simulink model "autosar_bsw_simulation"  (R2022b)
settings: Solver=VariableStepAuto  StartTime=0.0  StopTime=10.0  RelTol=1e-3
libraries: autosarlibdem x1, autosarlibnvm x1, simulink x1
settings Model: Creator=The MathWorks, Inc.  LastModifiedBy=The MathWorks, Inc.
settings SolverCC: AlgebraicLoopSolver=TrustRegion
settings DataIOCC: ReturnWorkspaceOutputs=off
settings DebuggingCC: UnconnectedInputMsg=warning  UnconnectedOutputMsg=warning  UnconnectedLineMsg=warning  PregeneratedLibrarySubsystemCodeDiagnostic=none  SFMachineParentedDataDiag=warning  ArithmeticOperatorsInVariantConditions=warning
settings ModelReferenceCC: EnableRefExpFcnMdlSchedulingChecks=on
settings SFSimCC: SimUseLocalCustomCode=off  CustomCodeUndefinedFunction=UseInterfaceOnly
settings RTWCC: RTWUseLocalCustomCode=off

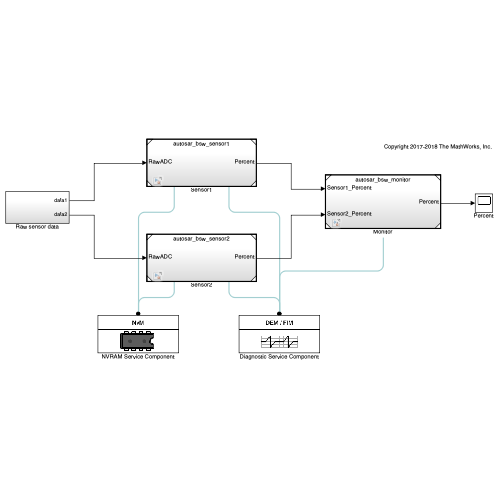
[thumbnail: Simulink's stored preview of the top-level diagram]
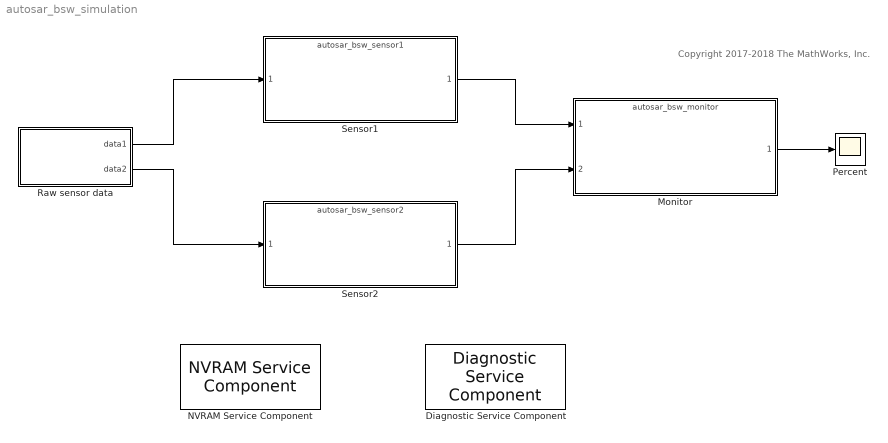
== system autosar_bsw_simulation ==
  note: Copyright 2017-2018 The MathWorks, Inc.
  Diagnostic Service Component : autosarlibdem/Diagnostic Service Component  ClientPortNames={'S1StuckHigh', 'S1StuckLow', 'S2StuckHigh', 'S2StuckLow', 'TPS', 'TPS1StuckHigh', 'TPS1StuckLow', 'TPS2StuckHigh', 'TPS2StuckLow'}  ClientPortPortDefinedArguments={'1', '2', '3', '4', '5', '1', '2', '3', '4'}  MaxEventId=10  MaxFID=10  DemDebounceCounterIncrementStepSize=1  DemDebounceCounterDecrementStepSize=1  DemDebounceCounterFailedThreshold=2  DemDebounceCounterPassedThreshold=-1  InhibitionMatrix=zeros(11,'uint8')  EnableConditionIndexes=zeros(257,'uint8')  StorageConditionIndexes=zeros(257,'uint8')
  Monitor : ModelReference  ModelNameDialog=autosar_bsw_monitor.slx  SimulationMode=Normal  ModelReferenceVersion=7.0
  NVRAM Service Component : autosarlibnvm/NVRAM Service Component  ClientPortNames={'S1LowSetPoint', 'S2LowSetPoint'}  ClientPortPortDefinedArguments={'1', '2'}  MaxBlockId=10  NvInitValues={'0'}
  Percent : Scope
  Raw sensor data : Subsystem
  Sensor1 : ModelReference  ModelNameDialog=autosar_bsw_sensor1.slx  SimulationMode=Normal  ModelReferenceVersion=7.0
  Sensor2 : ModelReference  ModelNameDialog=autosar_bsw_sensor2.slx  SimulationMode=Normal  ModelReferenceVersion=7.0
  wires:
  Monitor/1 -> Percent/1
  Sensor2/1 -> Monitor/2
  Sensor1/1 -> Monitor/1
  Raw sensor data/1(data1) -> Sensor1/1
  Raw sensor data/2(data2) -> Sensor2/1

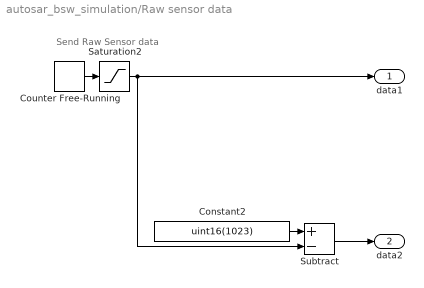
== system autosar_bsw_simulation/Raw sensor data ==
  note: Send Raw Sensor data
  Constant2 : Constant  Value=uint16(1023)
  Counter Free-Running : simulink/Sources/Counter Free-Running  NumBits=16  tsamp=.005
  Saturation2 : Saturate  UpperLimit=1023  LowerLimit=0  LinearizeAsGain=off  ZeroCross=off  OutDataTypeStr=uint16
  Subtract : Sum  Inputs=+-
  data1 : Outport  VectorParamsAs1DForOutWhenUnconnected=off
  data2 : Outport  Port=2  VectorParamsAs1DForOutWhenUnconnected=off
  wires:
  Constant2/1 -> Subtract/1
  Counter Free-Running/1 -> Saturation2/1
  Subtract/1 -> data2/1
  Saturation2/1 -> data1/1, Subtract/2
